simulink library "variableFlowProfileCalculation_ul"  (R2018b)
settings: Solver=VariableStepAuto  StartTime=0.0  StopTime=10.0  RelTol=1e-3
libraries: dspmtrx3 x6, simulink x3
settings Model: Creator=James Reed  LastModifiedBy=James Reed

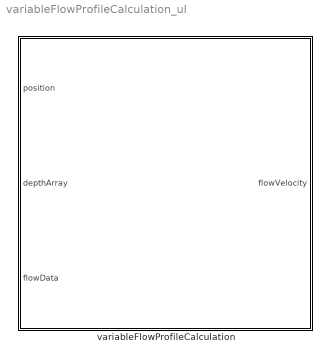
== system variableFlowProfileCalculation_ul ==
  variableFlowProfileCalculation : Subsystem

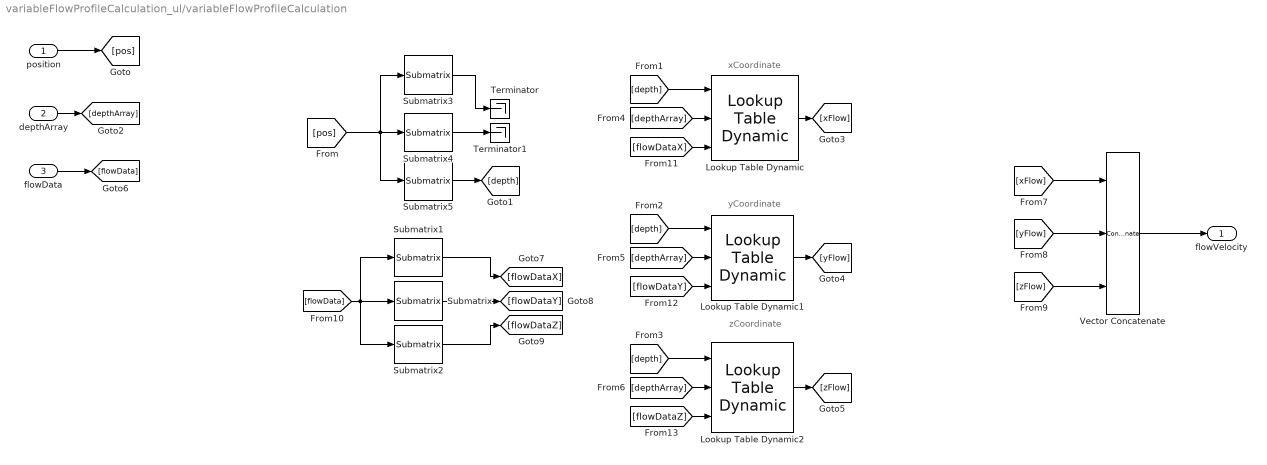
== system variableFlowProfileCalculation_ul/variableFlowProfileCalculation ==
  note: xCoordinate
  note: zCoordinate
  note: yCoordinate
  "position " : Inport
  "depthArray " : Inport  Port=2
  "flowData " : Inport  Port=3
  Lookup Table Dynamic : simulink/Lookup Tables/Lookup Table Dynamic  LookUpMeth=Interpolation-Use End Values  OutDataType=fixdt('double')  OutScaling=[]  OutputDataTypeScalingMode=Specify via dialog  OutDataTypeStr=double  DoSatur=off
      settings: SourceProductName=Simulink
  Lookup Table Dynamic1 : simulink/Lookup Tables/Lookup Table Dynamic  LookUpMeth=Interpolation-Use End Values  OutDataType=fixdt('double')  OutScaling=[]  OutputDataTypeScalingMode=Specify via dialog  OutDataTypeStr=double  DoSatur=off
      settings: SourceProductName=Simulink
  Lookup Table Dynamic2 : simulink/Lookup Tables/Lookup Table Dynamic  LookUpMeth=Interpolation-Use End Values  OutDataType=fixdt('double')  OutScaling=[]  OutputDataTypeScalingMode=Specify via dialog  OutDataTypeStr=double  DoSatur=off
      settings: SourceProductName=Simulink
  Submatrix : dspmtrx3/Submatrix  RowSpan=One row  RowStartMode=Middle  RowStartIndex=1  RowEndMode=Last  RowEndIndex=1  ColSpan=All columns  ColStartMode=First  ColStartIndex=1  ColEndMode=Last  ColEndIndex=1
  Submatrix{1,3..5} (4 alike) : dspmtrx3/Submatrix  RowSpan=One row  RowStartMode=First  RowStartIndex=1  RowEndMode=Last  RowEndIndex=1  ColSpan=All columns  ColStartMode=First  ColStartIndex=1  ColEndMode=Last  ColEndIndex=1
  Submatrix2 : dspmtrx3/Submatrix  RowSpan=One row  RowStartMode=Last  RowStartIndex=1  RowEndMode=Last  RowEndIndex=1  ColSpan=All columns  ColStartMode=First  ColStartIndex=1  ColEndMode=Last  ColEndIndex=1
  Terminator : Terminator
  Terminator1 : Terminator
  Vector Concatenate : Concatenate  NumInputs=3  Mode=Multidimensional array
  "flowVelocity " : Outport
  wires:
  [depthArray] -> Lookup Table Dynamic1/2
  Submatrix2/1 -> [flowDataZ]
  [pos] -> Submatrix3/1, Submatrix5/1, Submatrix4/1
  [depthArray] -> Lookup Table Dynamic/2
  Lookup Table Dynamic2/1 -> [zFlow]
  Lookup Table Dynamic/1 -> [xFlow]
  Submatrix1/1 -> [flowDataX]
  Submatrix3/1 -> Terminator/1
  [flowData] -> Submatrix/1, Submatrix1/1, Submatrix2/1
  [flowDataZ] -> Lookup Table Dynamic2/3
  "depthArray "/1 -> [depthArray]
  Submatrix/1 -> [flowDataY]
  [depthArray] -> Lookup Table Dynamic2/2
  Submatrix5/1 -> [depth]
  "flowData "/1 -> [flowData]
  [depth] -> Lookup Table Dynamic/1
  [flowDataY] -> Lookup Table Dynamic1/3
  [depth] -> Lookup Table Dynamic2/1
  [yFlow] -> Vector Concatenate/2
  [flowDataX] -> Lookup Table Dynamic/3
  [xFlow] -> Vector Concatenate/1
  Lookup Table Dynamic1/1 -> [yFlow]
  Submatrix4/1 -> Terminator1/1
  [depth] -> Lookup Table Dynamic1/1
  Vector Concatenate/1 -> "flowVelocity "/1
  "position "/1 -> [pos]
  [zFlow] -> Vector Concatenate/3
